simulink model "Kalman_Beispiel_SRF02"  (R2019b)
settings: Solver=FixedStepDiscrete  StartTime=0.0  StopTime=Inf  FixedStep=0.1  RelTol=1e-3  EnableMultiTasking=on
undefined symbols (not defined in the file): Discrete, Time
libraries: ctrlSharedLib x1, realtime_pacer_lib x1, robotlib x1, simulink x1
settings Model: Creator=Student  LastModifiedBy=mackst
settings DataIOCC: ReturnWorkspaceOutputs=off
settings DebuggingCC: ArithmeticOperatorsInVariantConditions=warning
settings SFSimCC: SimUseLocalCustomCode=off  CustomCodeUndefinedFunction=UseInterfaceOnly
settings RTWCC: RTWUseLocalCustomCode=off

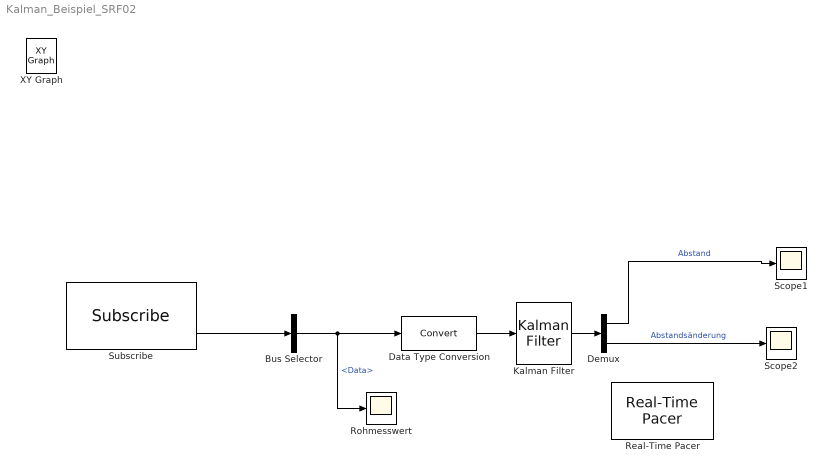
== system Kalman_Beispiel_SRF02 ==
  Bus Selector : BusSelector  OutputSignals=Data
  Data Type Conversion : DataTypeConversion
  Demux : Demux  Outputs=2
  Kalman Filter : ctrlSharedLib/Kalman Filter  TimeDomain=Discrete-Time  UseCurrentEstimator=on  ModelSource=Individual A, B, C, D matrices  ModelSourceVariable=ss(0.95,1,1,0,1)  A=[1 0.1;0 1]  B=0  C=[1 0]  D=0  NumberOfStates=1  NumberOfInputs=1  NumberOfOutputs=1  InitialEstimateSource=Dialog  X0=0  P0=10  UseK=off  UseGH=off  NumberOfProcessNoiseInputs=1  G=1  TimeInvariantG=on  H=0  TimeInvariantH=on  Q=[0.000025 0.0005; 0.0005 0.01]  TimeInvariantQ=on  R=0.0049  TimeInvariantR=on  N=0  TimeInvariantN=on  AddInputPort=off  AddEnablePort=off  OutputEstimatedY=off  OutputP=off  Ts=0.1
      settings: SourceProductBaseCode=CT
  Real-Time Pacer : realtime_pacer_lib/Real-Time Pacer  simTimePerRealTime=1
  Rohmesswert : Scope
  Scope1 : Scope
  Scope2 : Scope
  Subscribe : robotlib/Subscribe  topicSource=Select from ROS network  topic=/range_val  messageType=std_msgs/UInt16  sampleTime=-1  messageQueueLength=51
      settings: SourceProductName=ROS Toolbox
  XY Graph : simulink/Sinks/XY Graph  IOType=viewer  xmin=-1  xmax=1  ymin=-1  ymax=1  st=-1
  wires:
  Data Type Conversion/1 -> Kalman Filter/1
  Demux/2 -> Scope2/1  "Abstandsänderung"
  Demux/1 -> Scope1/1  "Abstand"
  Kalman Filter/1 -> Demux/1
  Bus Selector/1 -> Rohmesswert/1, Data Type Conversion/1  "<Data>"
  Subscribe/2 -> Bus Selector/1
